simulink model "test_link_demux_old"  (Simulink 7.0)
settings: Solver=ode45  StartTime=0.0  StopTime=25  RelTol=1e-3
libraries: xbsIndex_r4 x28, isi_correlator_lib x13, xps_library x9, casper_library x1
settings Model: Creator=wjm  LastModifiedBy=wjm

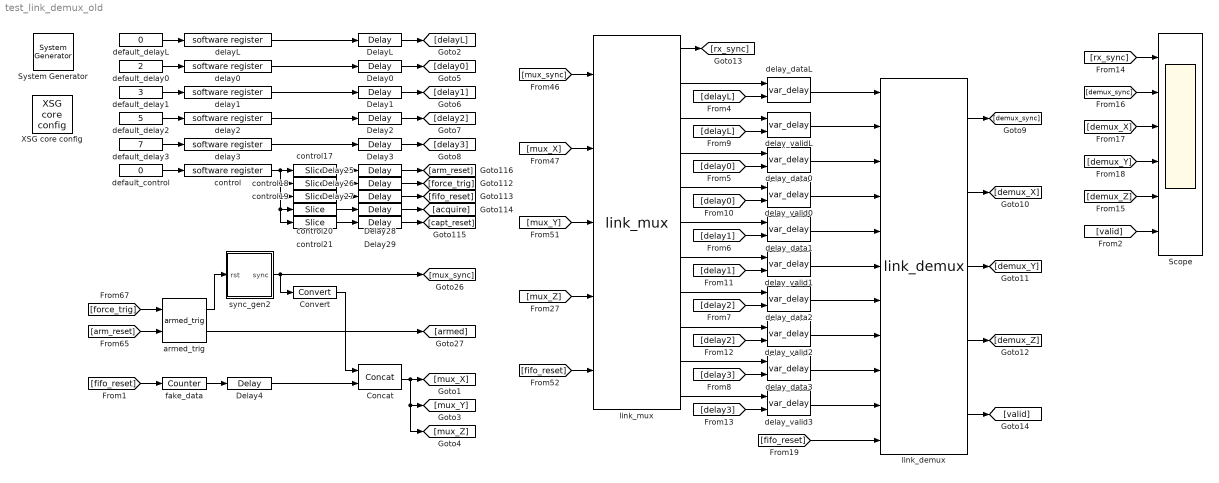
== system test_link_demux_old ==
  " System Generator" : xbsIndex_r4/ System Generator  Tag=genX  SystemSampleTime=-1  xilinxfamily=virtex5  part=xc5vsx95t  speed=-1  package=ff1136  synthesis_tool=XST  clock_wrapper=Clock Enables  directory=./isi_correlator_cropped/sysgen  testbench=off  simulink_period=1  sysclk_period=5  dcm_input_clock_period=100  incr_netlist=off  trim_vbits=Everywhere in SubSystem  dbl_ovrd=According to Block Masks  core_generation=According to Block Masks  run_coregen=off  deprecated_control=off  eval_field=0  block_type=sysgen
      settings: block_version=10.1.1
  Concat : xbsIndex_r4/Concat  num_inputs=2  dbl_ovrd=off  block_type=concat
      settings: block_version=10.1.3
  Convert : xbsIndex_r4/Convert  arith_type=Unsigned  n_bits=1  bin_pt=0  quantization=Truncate  overflow=Wrap  latency=0  dbl_ovrd=off  pipeline=off  block_type=convert
      settings: block_version=10.1.3
  Delay{0..3,25..29} (9 alike) : xbsIndex_r4/Delay  en=off  latency=3  dbl_ovrd=off  reg_retiming=off  block_type=delay
  Delay4 : xbsIndex_r4/Delay  en=off  latency=2  dbl_ovrd=off  reg_retiming=off  block_type=delay
  DelayL : xbsIndex_r4/Delay  en=off  latency=3  dbl_ovrd=off  reg_retiming=off  block_type=delay
  Scope : Scope  NumInputPorts=6
      settings: YMin=-5~-5~-5~-5~-5~-5  YMax=5~5~5~5~5~5  MaxDataPoints=2000
  XSG core config : xps_library/XSG core config  Tag=xps:xsg  SystemSampleTime=-1  hw_sys=ROACH:sx95t  ibob_linux=off  clk_src=adc0_clk  iBOB_clk_src=sys_clk  BEE2_ctrl_clk_src=sys_clk  BEE2_usr_clk_src=sys_clk  ROACH_clk_src=adc0_clk  CORR_clk_src=sys_clk  gpio_clk_io_group=iBOB:sma  gpio_clk_bit_index=0  clk_rate=200  sample_period=1  synthesis_tool=XST  mpc_type=powerpc440_ext
  armed_trig : isi_correlator_lib/armed_trig  SystemSampleTime=-1
  control : xps_library/software register  Tag=xps:sw_reg  SystemSampleTime=-1  io_dir=From Processor  arith_type=Unsigned  bitwidth=32  bin_pt=0  sample_period=1  gw_name=test_link_demux_old_control_user_data_out
      link override corr_3ghz_10_1_corr_id_user_data_out: arith_type=Unsigned  n_bits=32  bin_pt=0  period=1
      link override corr_3ghz_10_1_exp_corr_id_user_data_out: arith_type=Unsigned  n_bits=32  bin_pt=0  period=1
      link override isi_corr_eq_coeff_user_data_out: arith_type=Unsigned  n_bits=32  bin_pt=0  period=1
      link override isi_correlator_control_user_data_out: arith_type=Unsigned  n_bits=32  bin_pt=0  period=1
      link override isi_correlator_cropped_control_user_data_out: arith_type=Unsigned  n_bits=32  bin_pt=0  period=1
      link override isi_correlator_eq_coeff_user_data_out: arith_type=Unsigned  n_bits=32  bin_pt=0  period=1
      link override isi_spectrometer_control_user_data_out: arith_type=Unsigned  n_bits=32  bin_pt=0  period=1
      link override isi_spectrometer_cropped_control_user_data_out: arith_type=Unsigned  n_bits=32  bin_pt=0  period=1
      link override isi_spectrometer_with_pfb_control_user_data_out: arith_type=Unsigned  n_bits=32  bin_pt=0  period=1
      link override roach_spectrometer_control_user_data_out: arith_type=Unsigned  n_bits=32  bin_pt=0  period=1
      link override test_link_demux_control_user_data_out: arith_type=Unsigned  n_bits=32  bin_pt=0  period=1
      link override test_link_demux_old_control_user_data_out: arith_type=Unsigned  n_bits=32  bin_pt=0  period=1
  control17 : xbsIndex_r4/Slice  nbits=1  boolean_output=on  mode=Lower Bit Location + Width  bit1=0  base1=MSB of Input  bit0=0  base0=LSB of Input  dbl_ovrd=off  block_type=slice
      settings: infoedit="Extracts a given range of bits from each input sample and presents it at the output.  The output type is ordinarily unsigned with binary point at zero, but can be Boolean when the slice is one bit wide.<P><P>Hardware notes: In hardware this block costs nothing."  block_version=10.1.3
  control18 : xbsIndex_r4/Slice  nbits=1  boolean_output=on  mode=Lower Bit Location + Width  bit1=0  base1=MSB of Input  bit0=1  base0=LSB of Input  dbl_ovrd=off  block_type=slice
      settings: infoedit="Extracts a given range of bits from each input sample and presents it at the output.  The output type is ordinarily unsigned with binary point at zero, but can be Boolean when the slice is one bit wide.<P><P>Hardware notes: In hardware this block costs nothing."  block_version=10.1.3
  control19 : xbsIndex_r4/Slice  nbits=1  boolean_output=on  mode=Lower Bit Location + Width  bit1=0  base1=MSB of Input  bit0=2  base0=LSB of Input  dbl_ovrd=off  block_type=slice
      settings: infoedit="Extracts a given range of bits from each input sample and presents it at the output.  The output type is ordinarily unsigned with binary point at zero, but can be Boolean when the slice is one bit wide.<P><P>Hardware notes: In hardware this block costs nothing."  block_version=10.1.3
  control20 : xbsIndex_r4/Slice  nbits=1  boolean_output=on  mode=Lower Bit Location + Width  bit1=0  base1=MSB of Input  bit0=3  base0=LSB of Input  dbl_ovrd=off  block_type=slice
      settings: infoedit="Extracts a given range of bits from each input sample and presents it at the output.  The output type is ordinarily unsigned with binary point at zero, but can be Boolean when the slice is one bit wide.<P><P>Hardware notes: In hardware this block costs nothing."  block_version=10.1.3
  control21 : xbsIndex_r4/Slice  nbits=1  boolean_output=on  mode=Lower Bit Location + Width  bit1=0  base1=MSB of Input  bit0=4  base0=LSB of Input  dbl_ovrd=off  block_type=slice
      settings: infoedit="Extracts a given range of bits from each input sample and presents it at the output.  The output type is ordinarily unsigned with binary point at zero, but can be Boolean when the slice is one bit wide.<P><P>Hardware notes: In hardware this block costs nothing."  block_version=10.1.3
  default_control : Constant  Value=0  OutDataType=sfix(16)  OutScaling=2^0  SampleTime=1
  default_delay0 : Constant  Value=2  OutDataType=sfix(16)  OutScaling=2^0  SampleTime=1
  default_delay1 : Constant  Value=3  OutDataType=sfix(16)  OutScaling=2^0  SampleTime=1
  default_delay2 : Constant  Value=5  OutDataType=sfix(16)  OutScaling=2^0  SampleTime=1
  default_delay3 : Constant  Value=7  OutDataType=sfix(16)  OutScaling=2^0  SampleTime=1
  default_delayL : Constant  Value=0  OutDataType=sfix(16)  OutScaling=2^0  SampleTime=1
  delay0 : xps_library/software register  Tag=xps:sw_reg  SystemSampleTime=-1  io_dir=From Processor  arith_type=Unsigned  bitwidth=32  bin_pt=0  sample_period=1  gw_name=test_link_demux_old_delay0_user_data_out
      link override convert: arith_type=Unsigned  n_bits=32  bin_pt=0
      link override test_link_demux_delay0_user_data_out: arith_type=Unsigned  n_bits=32  bin_pt=0  period=1
      link override test_link_demux_old_delay0_user_data_out: arith_type=Unsigned  n_bits=32  bin_pt=0  period=1
  delay1 : xps_library/software register  Tag=xps:sw_reg  SystemSampleTime=-1  io_dir=From Processor  arith_type=Unsigned  bitwidth=32  bin_pt=0  sample_period=1  gw_name=test_link_demux_old_delay1_user_data_out
      link override convert: arith_type=Unsigned  n_bits=32  bin_pt=0
      link override test_link_demux_delay1_user_data_out: arith_type=Unsigned  n_bits=32  bin_pt=0  period=1
      link override test_link_demux_old_delay1_user_data_out: arith_type=Unsigned  n_bits=32  bin_pt=0  period=1
  delay2 : xps_library/software register  Tag=xps:sw_reg  SystemSampleTime=-1  io_dir=From Processor  arith_type=Unsigned  bitwidth=32  bin_pt=0  sample_period=1  gw_name=test_link_demux_old_delay2_user_data_out
      link override convert: arith_type=Unsigned  n_bits=32  bin_pt=0
      link override test_link_demux_delay2_user_data_out: arith_type=Unsigned  n_bits=32  bin_pt=0  period=1
      link override test_link_demux_old_delay2_user_data_out: arith_type=Unsigned  n_bits=32  bin_pt=0  period=1
  delay3 : xps_library/software register  Tag=xps:sw_reg  SystemSampleTime=-1  io_dir=From Processor  arith_type=Unsigned  bitwidth=32  bin_pt=0  sample_period=1  gw_name=test_link_demux_old_delay3_user_data_out
      link override convert: arith_type=Unsigned  n_bits=32  bin_pt=0
      link override test_link_demux_delay3_user_data_out: arith_type=Unsigned  n_bits=32  bin_pt=0  period=1
      link override test_link_demux_old_delay3_user_data_out: arith_type=Unsigned  n_bits=32  bin_pt=0  period=1
  delayL : xps_library/software register  Tag=xps:sw_reg  SystemSampleTime=-1  io_dir=From Processor  arith_type=Unsigned  bitwidth=32  bin_pt=0  sample_period=1  gw_name=test_link_demux_old_delayL_user_data_out
      link override convert: arith_type=Unsigned  n_bits=32  bin_pt=0
      link override test_link_demux_delayL_user_data_out: arith_type=Unsigned  n_bits=32  bin_pt=0  period=1
      link override test_link_demux_old_delayL_user_data_out: arith_type=Unsigned  n_bits=32  bin_pt=0  period=1
  delay_data{0..3} (4 alike) : isi_correlator_lib/var_delay  SystemSampleTime=-1
  delay_dataL : isi_correlator_lib/var_delay  SystemSampleTime=-1
  delay_valid{0..3} (4 alike) : isi_correlator_lib/var_delay  SystemSampleTime=-1
  delay_validL : isi_correlator_lib/var_delay  SystemSampleTime=-1
  fake_data : xbsIndex_r4/Counter  cnt_type=Free Running  cnt_to=Inf  operation=Up  start_count=0  cnt_by_val=1  arith_type=Unsigned  n_bits=31  bin_pt=0  load_pin=off  rst=on  en=off  explicit_period=on  period=1  dbl_ovrd=off  use_behavioral_HDL=off  use_rpm=off  implementation=Fabric  block_type=counter
  link_demux : isi_correlator_lib/link_demux  SystemSampleTime=-1  input_latency=1  hold_latency=1  align_latency=1  and_latency=1  or_latency=1  mux_latency=1
  link_mux : isi_correlator_lib/link_mux  SystemSampleTime=-1
  sync_gen2 : Subsystem  AncestorBlock=isi_correlator_lib/sync_gen2  mask(sync_gen2){using_pfb_fir=off, pfb_fir_taps=1, using_fft=off, fft_size=7, fft_inputs=4, fft_orders=[2 2 2 1], using_ct=off, ct_type=Double-buffered, using_vacc=off, vacc_length=0, using_scale_factor=on, scale_factor=2^9}
      mask prompts: using_pfb_fir "This design uses a PFB FIR."; pfb_fir_taps "Number of taps in PFB FIR:"; using_fft "This design uses an FFT."; fft_size "Size of FFT: (2^?)"; fft_inputs "Number of FFT inputs: (2^?)"; fft_orders "Order of FFT reorders: (vector)"; using_ct "This design uses a corner turner."; ct_type "Type of reorder operation:"; using_vacc "This design uses a vector accumulator."; vacc_length "Length of accumulations: (2^?)"; using_scale_factor "Scale the minimum period by an arbitrary amount."; scale_factor "Scale factor:"
      mask help: This block generates a sync pulse of an appropriate period based on the specified mask parameters.
      mask init:
      | sync_gen2_init(gcb, ...
      |     'using_pfb_fir', using_pfb_fir, ...
      |     'pfb_fir_taps', pfb_fir_taps, ...
      |     'using_fft', using_fft, ...
      |     'fft_size', fft_size, ...
      |     'fft_inputs', fft_inputs, ...
      |     'fft_orders', fft_orders, ...
      |     'using_ct', using_ct, ...
      |     'ct_type', ct_type, ...
      |     'using_vacc', using_vacc, ...
      |     'vacc_length', vacc_length, ...
      |     'using_scale_factor', using_scale_factor, ...
      |     'scale_factor', scale_factor);
      settings: AttributesFormatString=sync_period=512
      mask StyleString: checkbox,edit,checkbox,edit,edit,edit,checkbox,popup(Double-buffered|In-place),checkbox,edit,checkbox,edit
      mask CallbackString:
      | thisVariable = 'using_pfb_fir';
      | affectedVars = {'pfb_fir_taps'};
      | 
      | thisBlock = gcb();
      | thisVarState = get_param(thisBlock, thisVariable);
      | maskNames = get_param(thisBlock, 'MaskNames');
      | maskEnables = get_param(thisBlock, 'MaskEnables');
      | 
      | for varName = affectedVars
      |     varIndex = find(ismember(maskNames, varName));
      |     maskEnables{varIndex} = thisVarState;
      | end
      | 
      | set_param(thisBlock, 'MaskEnables', maskEnables);||thisVariable = 'using_fft';
      | affectedVars = {'fft_size', 'fft_inputs', 'fft_orders'};
      | 
      | thisBlock = gcb();
      | thisVarState = get_param(thisBlock, thisVariable);
      | maskNames = get_param(thisBlock, 'MaskNames');
      | maskEnables = get_param(thisBlock, 'MaskEnables');
      | 
      | for varName = affectedVars
      |     varIndex = find(ismember(maskNames, varName));
      |     maskEnables{varIndex} = thisVarState;
      | end
      | 
      | set_param(thisBlock, 'MaskEnables', maskEnables);||||thisVariable = 'using_ct';
      | affectedVars = {'ct_type'};
      | 
      | thisBlock = gcb();
      | thisVarState = get_param(thisBlock, thisVariable);
      | maskNames = get_param(thisBlock, 'MaskNames');
      | maskEnables = get_param(thisBlock, 'MaskEnables');
      | 
      | for varName = affectedVars
      |     varIndex = find(ismember(maskNames, varName));
      |     maskEnables{varIndex} = thisVarState;
      | end
      | 
      | set_param(thisBlock, 'MaskEnables', maskEnables);||thisVariable = 'using_vacc';
      | affectedVars = {'vacc_length'};
      | 
      | thisBlock = gcb();
      | thisVarState = get_param(thisBlock, thisVariable);
      | maskNames = get_param(thisBlock, 'MaskNames');
      | maskEnables = get_param(thisBlock, 'MaskEnables');
      | 
      | for varName = affectedVars
      |     varIndex = find(ismember(maskNames, varName));
      |     maskEnables{varIndex} = thisVarState;
      | end
      | 
      | set_param(thisBlock, 'MaskEnables', maskEnables);||thisVariable = 'using_scale_factor';
      | affectedVars = {'scale_factor'};
      | 
      | thisBlock = gcb();
      | thisVarState = get_param(thisBlock, thisVariable);
      | maskNames = get_param(thisBlock, 'MaskNames');
      | maskEnables = get_param(thisBlock, 'MaskEnables');
      | 
      | for varName = affectedVars
      |     varIndex = find(ismember(maskNames, varName));
      |     maskEnables{varIndex} = thisVarState;
      | end
      | 
      | set_param(thisBlock, 'MaskEnables', maskEnables);|
  wires:
  delay_dataL/1 -> link_demux/1
  delay_validL/1 -> link_demux/2
  delay_data0/1 -> link_demux/3
  delay_valid0/1 -> link_demux/4
  delay_data1/1 -> link_demux/5
  delay_valid1/1 -> link_demux/6
  delay_data2/1 -> link_demux/7
  delay_valid2/1 -> link_demux/8
  delay_data3/1 -> link_demux/9
  delay_valid3/1 -> link_demux/10
  link_mux/2 -> delay_dataL/1
  link_mux/3 -> delay_validL/1
  link_mux/4 -> delay_data0/1
  link_mux/5 -> delay_valid0/1
  link_mux/6 -> delay_data1/1
  link_mux/7 -> delay_valid1/1
  link_mux/8 -> delay_data2/1
  link_mux/9 -> delay_valid2/1
  link_mux/10 -> delay_data3/1
  link_mux/11 -> delay_valid3/1
  default_delayL/1 -> delayL/1
  delayL/1 -> DelayL/1
  default_delay0/1 -> delay0/1
  delay0/1 -> Delay0/1
  default_delay1/1 -> delay1/1
  delay1/1 -> Delay1/1
  default_delay2/1 -> delay2/1
  delay2/1 -> Delay2/1
  default_delay3/1 -> delay3/1
  delay3/1 -> Delay3/1
  [arm_reset] -> armed_trig/2
  armed_trig/1 -> sync_gen2/1(rst)
  armed_trig/2 -> [armed]
  sync_gen2/1(sync) -> [mux_sync], Convert/1
  control21/1 -> Delay29/1
  control20/1 -> Delay28/1
  control19/1 -> Delay27/1
  control18/1 -> Delay26/1
  control17/1 -> Delay25/1
  control/1 -> control17/1, control18/1, control19/1, control21/1, control20/1
  Delay26/1 -> [force_trig]
  Delay27/1 -> [fifo_reset]
  Delay28/1 -> [acquire]
  Delay29/1 -> [capt_reset]
  default_control/1 -> control/1
  Delay25/1 -> [arm_reset]
  [fifo_reset] -> fake_data/1
  fake_data/1 -> Delay4/1
  [mux_sync] -> link_mux/1
  [mux_X] -> link_mux/2
  [mux_Y] -> link_mux/3
  [mux_Z] -> link_mux/4
  [fifo_reset] -> link_mux/5
  DelayL/1 -> [delayL]
  Delay0/1 -> [delay0]
  Delay1/1 -> [delay1]
  Delay2/1 -> [delay2]
  Delay3/1 -> [delay3]
  [delayL] -> delay_dataL/2
  [delayL] -> delay_validL/2
  [delay0] -> delay_data0/2
  [delay0] -> delay_valid0/2
  [delay1] -> delay_data1/2
  [delay1] -> delay_valid1/2
  [delay2] -> delay_data2/2
  [delay2] -> delay_valid2/2
  [delay3] -> delay_data3/2
  [delay3] -> delay_valid3/2
  link_demux/1 -> [demux_sync]
  link_demux/2 -> [demux_X]
  link_demux/3 -> [demux_Y]
  link_demux/4 -> [demux_Z]
  link_mux/1 -> [rx_sync]
  [rx_sync] -> Scope/1
  [demux_sync] -> Scope/2
  [demux_X] -> Scope/3
  [demux_Y] -> Scope/4
  [demux_Z] -> Scope/5
  [force_trig] -> armed_trig/1
  [fifo_reset] -> link_demux/11
  Delay4/1 -> Concat/2
  Convert/1 -> Concat/1
  Concat/1 -> [mux_X], [mux_Z], [mux_Y]
  link_demux/5 -> [valid]
  [valid] -> Scope/6

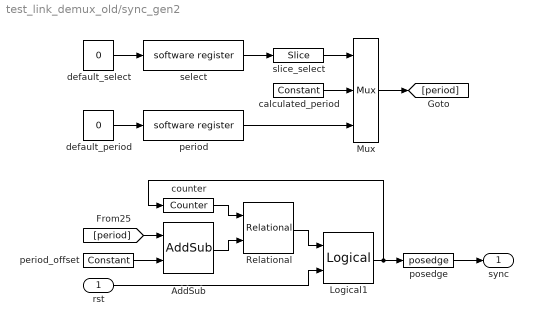
== system test_link_demux_old/sync_gen2 ==
  rst : Inport  OutDataType=sfix(16)  OutScaling=2^0
  AddSub : xbsIndex_r4/AddSub  mode=Subtraction  use_carryin=off  use_carryout=off  en=off  latency=2  precision=Full  arith_type=Unsigned  n_bits=16  bin_pt=14  quantization=Truncate  overflow=Wrap  dbl_ovrd=off  use_behavioral_HDL=off  pipelined=off  use_rpm=on  hw_selection=Fabric  block_type=addsub
      settings: block_version=10.1.3
  Logical1 : xbsIndex_r4/Logical  logical_function=OR  inputs=2  en=off  latency=0  precision=Full  arith_type=Unsigned  n_bits=16  bin_pt=0  align_bp=on  dbl_ovrd=off  block_type=logical
  Mux : xbsIndex_r4/Mux  inputs=2  en=off  latency=0  precision=Full  arith_type=Unsigned  n_bits=16  bin_pt=14  quantization=Truncate  overflow=Wrap  dbl_ovrd=off  block_type=mux
  Relational : xbsIndex_r4/Relational  mode=a>=b  en=off  latency=1  dbl_ovrd=off  block_type=relational
      settings: block_version=10.1.3
  calculated_period : xbsIndex_r4/Constant  arith_type=Unsigned  const=512  n_bits=32  bin_pt=0  explicit_period=on  period=1  equ=P=C  opselect=C  inp2=PCIN>>17  opr=+  inp1=P  carry=CIN  dbl_ovrd=off  block_type=constant
      settings: block_version=10.1.1
  counter : xbsIndex_r4/Counter  cnt_type=Free Running  cnt_to=Inf  operation=Up  start_count=0  cnt_by_val=1  arith_type=Unsigned  n_bits=32  bin_pt=0  load_pin=off  rst=on  en=off  explicit_period=on  period=1  dbl_ovrd=off  use_behavioral_HDL=off  use_rpm=off  implementation=Fabric  block_type=counter
  default_period : Constant  Value=0  OutDataType=sfix(16)  OutScaling=2^0  SampleTime=1
  default_select : Constant  Value=0  OutDataType=sfix(16)  OutScaling=2^0  SampleTime=1
  period : xps_library/software register  Tag=xps:sw_reg  SystemSampleTime=-1  io_dir=From Processor  arith_type=Unsigned  bitwidth=32  bin_pt=0  sample_period=1  gw_name=isi_correlator_lib_sync_gen2_period_user_data_out
  period_offset : xbsIndex_r4/Constant  arith_type=Unsigned  const=3  n_bits=32  bin_pt=0  explicit_period=on  period=1  equ=P=C  opselect=C  inp2=PCIN>>17  opr=+  inp1=P  carry=CIN  dbl_ovrd=off  block_type=constant
      settings: block_version=10.1.1
  posedge : casper_library/Misc/posedge  Tag=Rising Edge Detector  SystemSampleTime=-1
  select : xps_library/software register  Tag=xps:sw_reg  SystemSampleTime=-1  io_dir=From Processor  arith_type=Unsigned  bitwidth=32  bin_pt=0  sample_period=1  gw_name=isi_correlator_lib_sync_gen2_select_user_data_out
  slice_select : xbsIndex_r4/Slice  nbits=1  boolean_output=on  mode=Lower Bit Location + Width  bit1=0  base1=MSB of Input  bit0=0  base0=LSB of Input  dbl_ovrd=off  block_type=slice
      settings: infoedit="Extracts a given range of bits from each input sample and presents it at the output.  The output type is ordinarily unsigned with binary point at zero, but can be Boolean when the slice is one bit wide.<P><P>Hardware notes: In hardware this block costs nothing."  block_version=10.1.3
  sync : Outport  OutDataType=sfix(16)  OutScaling=2^0
  wires:
  Mux/1 -> [period]
  period/1 -> Mux/3
  calculated_period/1 -> Mux/2
  slice_select/1 -> Mux/1
  default_period/1 -> period/1
  select/1 -> slice_select/1
  default_select/1 -> select/1
  [period] -> AddSub/1
  period_offset/1 -> AddSub/2
  AddSub/1 -> Relational/2
  counter/1 -> Relational/1
  Logical1/1 -> posedge/1, counter/1
  posedge/1 -> sync/1
  Relational/1 -> Logical1/1
  rst/1 -> Logical1/2
